simulink model "mcb_pmsm_foc_host_model_dyno_f28069m_Lab_2_GITHUB"  (R2023b)
settings: Solver=ode3  StartTime=0.0  StopTime=inf  RelTol=1e-3
undefined symbols (not defined in the file): PU_System_motor1, PU_System_motor2, Ts
libraries: instrumentseriallib x3, simulink x3, demo_controls x1
settings Model: Creator=The MathWorks, Inc.  LastModifiedBy=Jonathan
settings SolverCC: AlgebraicLoopSolver=TrustRegion  AutoInsertRateTranBlk=on  MaxZcPerStep=1
settings DataIOCC: LimitDataPoints=on  SaveFormat=Array  ReturnWorkspaceOutputs=off
settings OptimizationCC: LifeSpan=1  EfficientTunableParamExpr=on
settings DebuggingCC: UnderspecifiedInitializationDetection=Classic  MergeDetectMultiDrivingBlocksExec=none  SolverPrmCheckMsg=warning  ParameterPrecisionLossMsg=none  UnconnectedInputMsg=warning  UnconnectedOutputMsg=warning  UnconnectedLineMsg=warning  AllowSymbolicDim=off  PregeneratedLibrarySubsystemCodeDiagnostic=none  SFUnexpectedBacktrackingDiag=warning  SFNoUnconditionalDefaultTransitionDiag=warning  SFExecutionAtInitializationDiag=none  ArithmeticOperatorsInVariantConditions=warning
settings HardwareCC: ProdBitPerPointer=32  ProdLargestAtomicFloat=None  ProdIntDivRoundTo=Undefined  ProdEndianess=Unspecified  ProdWordSize=32  ProdHWDeviceType=32-bit Generic
settings ModelReferenceCC: EnableRefExpFcnMdlSchedulingChecks=on  PropagateSignalLabelsOutOfModel=off
settings SFSimCC: SimUseLocalCustomCode=off  MATLABDynamicMemAlloc=off
settings RTWCC: Description=Real-Time Workshop Embedded Coder  SystemTargetFile=ert.tlc  TemplateMakefile=ert_default_tmf  GenerateReport=on  RTWUseLocalCustomCode=off  IncludeHyperlinkInReport=on  LaunchReport=on  GenerateTraceInfo=on  GenerateTraceReport=on  GenerateTraceReportSl=on  GenerateTraceReportSf=on  GenerateTraceReportEml=on  DLArmComputeVersion=19.05
settings CodeAppCC: IgnoreCustomStorageClasses=off  StateflowObjectComments=on  InternalIdentifier=Classic
settings ERTTargetCC: MultiwordLength=2048  GenerateSampleERTMain=on  ERTCustomFileTemplate=example_file_process.tlc  ConvertIfToSwitch=off  SuppressUnreachableDefaultCases=off
settings ConfigComp: CovMetricSettings=dw  CovSaveCumulativeToWorkspaceVar=on  CovSaveSingleToWorkspaceVar=on  CovExternalEMLEnable=off  CovSFcnEnable=off

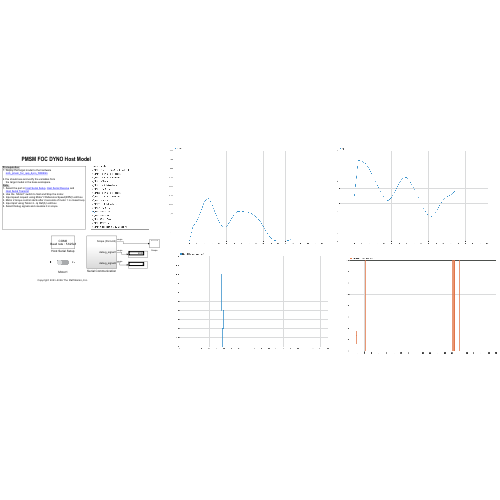
[thumbnail: Simulink's stored preview of the top-level diagram]
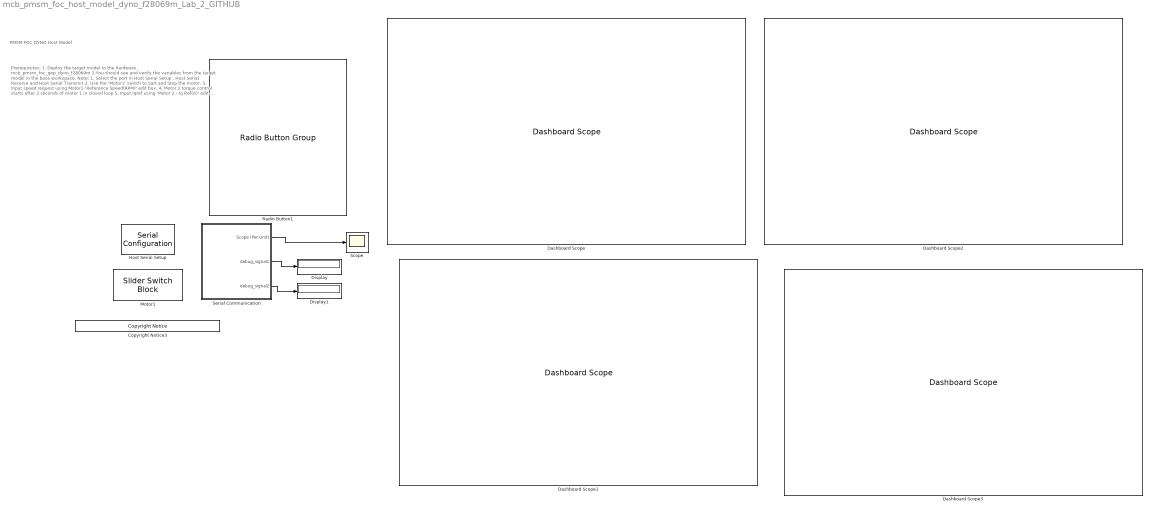
== system mcb_pmsm_foc_host_model_dyno_f28069m_Lab_2_GITHUB ==
  note: Prerequisites:
      | 1. Deploy the target model to the hardware
      | mcb_pmsm_foc_qep_dyno_f28069m
      |
      | 2.You should see and verify the variables from
      | the target model in the base workspace.
      | Note:
      | 1. Select the port in Host Serial Setup , Host Serial Receive and
      | Host Serial Transmit
      | 2. Use the 'Motor1' switch to Sart and Stop the motor.
      | 3. Input speed request using Motor1-'Reference Speed(RPM)' edit box.
      | 4. Motor 2 torque control starts after 2 seconds of motor 1 in closed loop
      | 5. Input Iqref using 'Motor 2 - Iq Ref(A)' edit box
      | 6. Select Debug signals and visualize it in scope.
  note: PMSM FOC DYNO Host Model
  Copyright Notice3 : demo_controls/Copyright Notice  year=2021  prod=tic2000
  Dashboard Scope : DashboardScope  TimeSpan=40  Ymin=-10  Ymax=5000  ScaleAtStop=off
  Dashboard Scope1 : DashboardScope  TimeSpan=100  Ymin=-0  Ymax=5  ScaleAtStop=off
  Dashboard Scope2 : DashboardScope  TimeSpan=40  Ymin=-6  Ymax=6  ScaleAtStop=off
  Dashboard Scope3 : DashboardScope  TimeSpan=40  Ymin=0  Ymax=4000  ScaleAtStop=off
  Display : Display
  Display1 : Display
  Host Serial Setup : instrumentseriallib/Serial Configuration  Priority=-99  PortSel=COM6  Port=COM6  ComPort=COM6  BaudRate=5.625e6  DataBits=8  Parity=none  StopBits=1  ByteOrder=little-endian  FlowControl=none  Timeout=2  SimulateUsing=Interpreted execution  BlockInModel=on  aMode=5
  Motor1 : SliderSwitchBlock  LabelPosition=Hide
      settings: Values={{'Stop', 'Start'}, [0 1]}
  Radio Button1 : RadioButtonGroup  LabelPosition=Hide  SelectedLabel=Mtr1&Mtr2: Pm  ButtonGroupName=Debug signals
      settings: Values={{'Mtr1: Speed ref & Speed feedback', 'Mtr1: Id ref & Id feedback', 'Mtr1: Iq ref & Iq feedback', 'Mtr1: Vd & Vq', 'Mtr1: Ia & Ib feedback', 'Mtr1: Pm & Te', 'Mtr2: Id ref & Id feedback', 'Mtr2: Iq ref & Iq feedback', 'Mtr2: Vd & Vq', 'Mtr2: Ia & Ib feedback', 'Mtr2: Pm & Te', 'Mtr1&Mtr2: Pm', 'Mtr1&Mtr2: Te', 'Mtr1&Mtr2: Pos', 'Mtr1&Mtr2: Ia', 'Mtr1 Speed ref & Mtr2 Speed fb'}, [1 2 3 4 5 6 7 8 9 10 11 12 13 14 15 0]}
  Scope : Scope
  Serial Communication : Subsystem
  wires:
  Serial Communication/1(Scope (Per-Unit)) -> Scope/1
  Serial Communication/2(debug_signal1) -> Display/1
  Serial Communication/3(debug_signal2) -> Display1/1

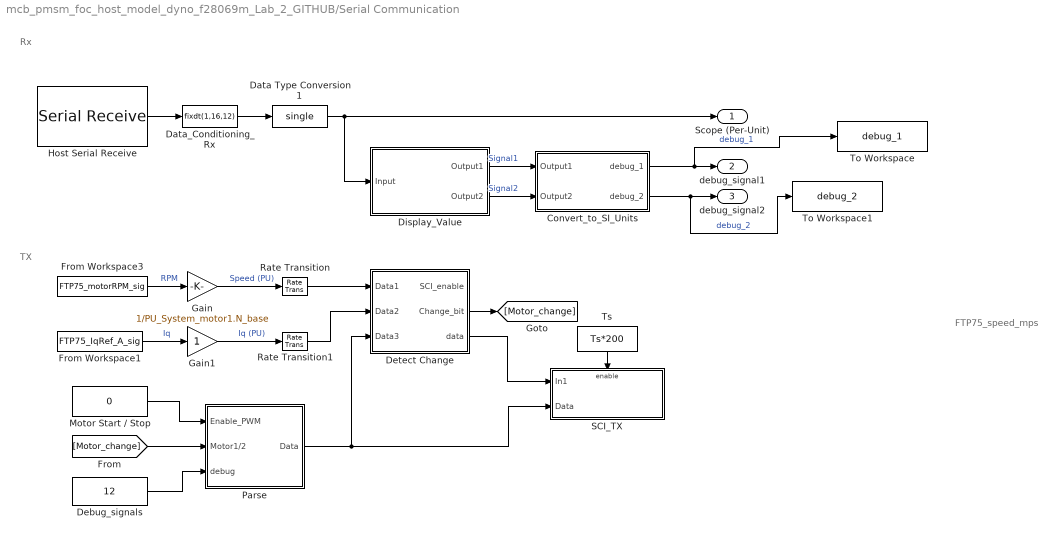
== system mcb_pmsm_foc_host_model_dyno_f28069m_Lab_2_GITHUB/Serial Communication ==
  note: FTP75_speed_mps
  note: TX
  note: Rx
  Convert_to_SI_Units : Subsystem
  Data Type Conversion1 : DataTypeConversion  OutDataTypeStr=single  RndMeth=Simplest  SaturateOnIntegerOverflow=off
  Data_Conditioning_Rx : DataTypeConversion  OutDataTypeStr=fixdt(1,16,12)  ConvertRealWorld=Stored Integer (SI)  RndMeth=Nearest
  Debug_signals : Constant  Value=12  OutDataTypeStr=uint16  SampleTime=0.03
  Detect Change : Subsystem
  Display_Value : MATLAB Function  TreatAsAtomicUnit=on
  From Workspace1 : FromWorkspace  VariableName=FTP75_IqRef_A_sig
  From Workspace3 : FromWorkspace  VariableName=FTP75_motorRPM_sig
  Gain : Gain  Gain=1/PU_System_motor1.N_base  OutDataTypeStr=single  RndMeth=Simplest
  Gain1 : Gain  RndMeth=Simplest  OutDataTypeStr=Inherit: Same as input
  Host Serial Receive : instrumentseriallib/Serial Receive  PortSel=COM6  Port=COM6  ComPort=COM6  DataType=uint16  SaveDataType=uint8  ToggleHeader=on  Header='SS'  DataSize=[600 2]  ToggleTerminator=on  Terminator=Custom terminator  CustomTerminator='EE'  InputFormat=Row major  ToggleDataSize=on  EnableBlockingMode=on  ActionDataUnavailable=Output last received value  ActionWhenDataUnavailable=Output last received value  CustomValue=0  SampleTime=Ts*200  SimulateUsing=Interpreted execution  BlockInModel=on  aMode=5
  Motor Start / Stop : Constant  Value=0  VectorParams1D=off  OutDataTypeStr=uint16  SampleTime=0.03
  Parse : Subsystem
  Rate Transition : RateTransition  OutPortSampleTime=0.03
  Rate Transition1 : RateTransition  OutPortSampleTime=0.03
  SCI_TX : Subsystem  TreatAsAtomicUnit=on
  To Workspace : ToWorkspace  VariableName=debug_1  SaveFormat=Timeseries  SampleTime=-1
  To Workspace1 : ToWorkspace  VariableName=debug_2  SaveFormat=Timeseries  SampleTime=-1
  Ts : Constant  Value=Ts*200  VectorParams1D=off  OutDataTypeStr=boolean  SampleTime=0.03
  Scope (Per-Unit) : Outport
  debug_signal1 : Outport  Port=2
  debug_signal2 : Outport  Port=3
  wires:
  Detect Change/2(Change_bit) -> [Motor_change]
  Gain/1 -> Rate Transition/1  "Speed (PU)"
  Motor Start / Stop/1 -> Parse/1(Enable_PWM)
  Parse/1(Data) -> SCI_TX/2(Data), Detect Change/3(Data3)
  Debug_signals/1 -> Parse/3(debug)
  Detect Change/3(data) -> SCI_TX/1(In1)
  Rate Transition1/1 -> Detect Change/2(Data2)
  Gain1/1 -> Rate Transition1/1  "Iq (PU)"
  Rate Transition/1 -> Detect Change/1(Data1)
  [Motor_change] -> Parse/2(Motor1/2)
  Host Serial Receive/1 -> Data_Conditioning_Rx/1
  Convert_to_SI_Units/2(debug_2) -> To Workspace1/1, debug_signal2/1  "debug_2"
  Convert_to_SI_Units/1(debug_1) -> To Workspace/1, debug_signal1/1  "debug_1"
  Data_Conditioning_Rx/1 -> Data Type Conversion1/1
  Display_Value/2(Output2) -> Convert_to_SI_Units/2(Output2)  "Signal2"
  Display_Value/1(Output1) -> Convert_to_SI_Units/1(Output1)  "Signal1"
  Data Type Conversion1/1 -> Scope (Per-Unit)/1, Display_Value/1(Input)
  Ts/1 -> SCI_TX/Enable
  From Workspace3/1 -> Gain/1  "RPM"
  From Workspace1/1 -> Gain1/1  "Iq"

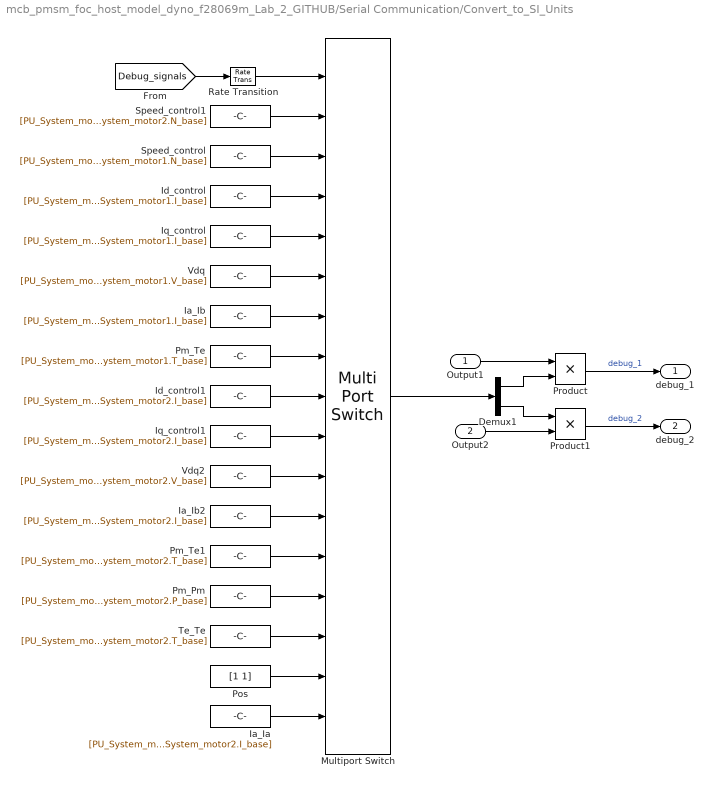
== system mcb_pmsm_foc_host_model_dyno_f28069m_Lab_2_GITHUB/Serial Communication/Convert_to_SI_Units ==
  Output1 : Inport
  Output2 : Inport  Port=2
  Demux1 : Demux  Outputs=2
  Ia_Ia : Constant  Value=[PU_System_motor1.I_base PU_System_motor2.I_base]  OutDataTypeStr=uint16  SampleTime=-1
  Ia_Ib : Constant  Value=[PU_System_motor1.I_base PU_System_motor1.I_base]  OutDataTypeStr=uint16  SampleTime=-1
  Ia_Ib2 : Constant  Value=[PU_System_motor2.I_base PU_System_motor2.I_base]  OutDataTypeStr=uint16  SampleTime=-1
  Id_control : Constant  Value=[PU_System_motor1.I_base PU_System_motor1.I_base]  OutDataTypeStr=uint16  SampleTime=-1
  Id_control1 : Constant  Value=[PU_System_motor2.I_base PU_System_motor2.I_base]  OutDataTypeStr=uint16  SampleTime=-1
  Iq_control : Constant  Value=[PU_System_motor1.I_base PU_System_motor1.I_base]  OutDataTypeStr=uint16  SampleTime=-1
  Iq_control1 : Constant  Value=[PU_System_motor2.I_base PU_System_motor2.I_base]  OutDataTypeStr=uint16  SampleTime=-1
  Multiport Switch : MultiPortSwitch  DataPortOrder=Zero-based contiguous  Inputs=16  DiagnosticForDefault=Warning  zeroidx=on  OutDataTypeStr=uint16  RndMeth=Simplest  SaturateOnIntegerOverflow=off  InputSameDT=off
  Pm_Pm : Constant  Value="[PU_System_motor1.P_base  PU_System_motor2.P_base]"  OutDataTypeStr=uint16  SampleTime=-1
  Pm_Te : Constant  Value="[PU_System_motor1.P_base  PU_System_motor1.T_base]"  OutDataTypeStr=uint16  SampleTime=-1
  Pm_Te1 : Constant  Value="[PU_System_motor2.P_base  PU_System_motor2.T_base]"  OutDataTypeStr=uint16  SampleTime=-1
  Pos : Constant  Value=[1 1]  OutDataTypeStr=uint16  SampleTime=-1
  Product : Product
  Product1 : Product
  Rate Transition : RateTransition  Deterministic=off
  Speed_control : Constant  Value=[PU_System_motor1.N_base PU_System_motor1.N_base]  OutDataTypeStr=uint16  SampleTime=-1
  Speed_control1 : Constant  Value=[PU_System_motor1.N_base PU_System_motor2.N_base]  OutDataTypeStr=uint16  SampleTime=-1
  Te_Te : Constant  Value="[PU_System_motor1.T_base  PU_System_motor2.T_base]"  OutDataTypeStr=uint16  SampleTime=-1
  Vdq : Constant  Value=[PU_System_motor1.V_base PU_System_motor1.V_base]  OutDataTypeStr=uint16  SampleTime=-1
  Vdq2 : Constant  Value=[PU_System_motor2.V_base PU_System_motor2.V_base]  OutDataTypeStr=uint16  SampleTime=-1
  debug_1 : Outport
  debug_2 : Outport  Port=2
  wires:
  Product/1 -> debug_1/1  "debug_1"
  Product1/1 -> debug_2/1  "debug_2"
  [Debug_signals] -> Rate Transition/1
  Multiport Switch/1 -> Demux1/1
  Demux1/1 -> Product/2
  Output1/1 -> Product/1
  Rate Transition/1 -> Multiport Switch/1
  Pos/1 -> Multiport Switch/16
  Ia_Ia/1 -> Multiport Switch/17
  Te_Te/1 -> Multiport Switch/15
  Pm_Pm/1 -> Multiport Switch/14
  Pm_Te1/1 -> Multiport Switch/13
  Ia_Ib2/1 -> Multiport Switch/12
  Vdq2/1 -> Multiport Switch/11
  Iq_control1/1 -> Multiport Switch/10
  Id_control1/1 -> Multiport Switch/9
  Pm_Te/1 -> Multiport Switch/8
  Ia_Ib/1 -> Multiport Switch/7
  Vdq/1 -> Multiport Switch/6
  Iq_control/1 -> Multiport Switch/5
  Id_control/1 -> Multiport Switch/4
  Speed_control/1 -> Multiport Switch/3
  Speed_control1/1 -> Multiport Switch/2
  Demux1/2 -> Product1/1
  Output2/1 -> Product1/2

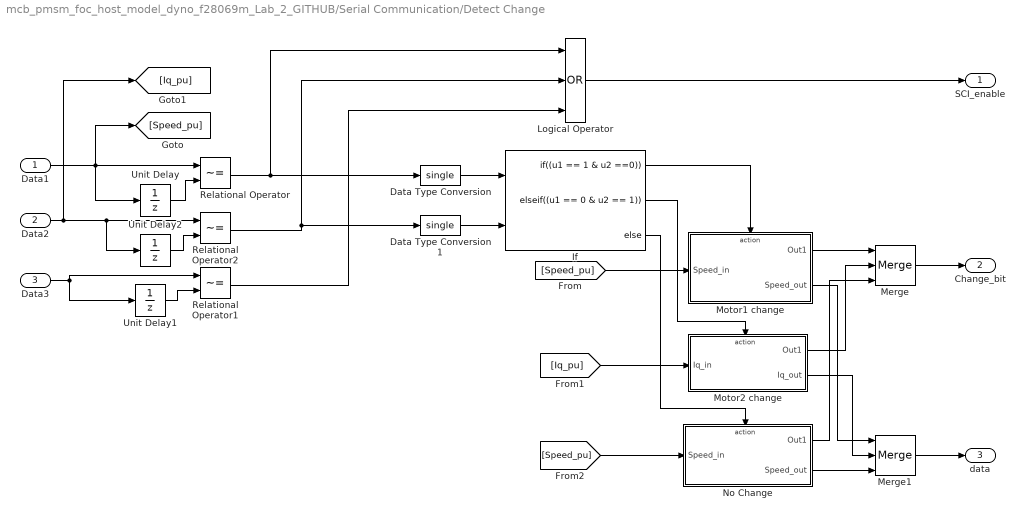
== system mcb_pmsm_foc_host_model_dyno_f28069m_Lab_2_GITHUB/Serial Communication/Detect Change ==
  Data1 : Inport
  Data2 : Inport  Port=2
  Data3 : Inport  Port=3
  Data Type Conversion : DataTypeConversion  OutDataTypeStr=single  SaturateOnIntegerOverflow=off  RndMeth=Floor
  Data Type Conversion1 : DataTypeConversion  OutDataTypeStr=single  SaturateOnIntegerOverflow=off  RndMeth=Floor
  If : If  NumInputs=2  IfExpression=(u1 == 1 & u2 ==0)  ElseIfExpressions=(u1 == 0 & u2 == 1)
  Logical Operator : Logic  Operator=OR  Inputs=3  AllPortsSameDT=off  OutDataTypeStr=boolean
  Merge : Merge  Inputs=3
  Merge1 : Merge  Inputs=3
  Motor1 change : Subsystem  TreatAsAtomicUnit=on
  Motor2 change : Subsystem  TreatAsAtomicUnit=on
  No Change : Subsystem  TreatAsAtomicUnit=on
  Relational Operator : RelationalOperator  Operator=~=  OutDataTypeStr=boolean  InputSameDT=off
  Relational Operator1 : RelationalOperator  Operator=~=  OutDataTypeStr=boolean  InputSameDT=off
  Relational Operator2 : RelationalOperator  Operator=~=  OutDataTypeStr=boolean  InputSameDT=off
  Unit Delay : UnitDelay  InitialCondition=0.5  SampleTime=-1  HasFrameUpgradeWarning=on
  Unit Delay1 : UnitDelay  SampleTime=-1  HasFrameUpgradeWarning=on
  Unit Delay2 : UnitDelay  InitialCondition=0.5  SampleTime=-1  HasFrameUpgradeWarning=on
  SCI_enable : Outport
  Change_bit : Outport  Port=2
  data : Outport  Port=3
  wires:
  Data1/1 -> [Speed_pu], Unit Delay/1, Relational Operator/1
  Unit Delay/1 -> Relational Operator/2
  Unit Delay2/1 -> Relational Operator2/2
  Data2/1 -> [Iq_pu], Unit Delay2/1, Relational Operator2/1
  Data3/1 -> Relational Operator1/1, Unit Delay1/1
  Logical Operator/1 -> SCI_enable/1
  Relational Operator2/1 -> Logical Operator/2, Data Type Conversion1/1
  Merge/1 -> Change_bit/1
  Relational Operator/1 -> Logical Operator/1, Data Type Conversion/1
  Motor2 change/1(Out1) -> Merge/2
  If/3 -> No Change/Action
  If/2 -> Motor2 change/Action
  No Change/1(Out1) -> Merge/3
  Merge1/1 -> data/1
  Motor2 change/2(Iq_out) -> Merge1/2
  No Change/2(Speed_out) -> Merge1/3
  Motor1 change/1(Out1) -> Merge/1
  Motor1 change/2(Speed_out) -> Merge1/1
  Data Type Conversion/1 -> If/1
  Data Type Conversion1/1 -> If/2
  If/1 -> Motor1 change/Action
  Unit Delay1/1 -> Relational Operator1/2
  Relational Operator1/1 -> Logical Operator/3
  [Speed_pu] -> Motor1 change/1(Speed_in)
  [Iq_pu] -> Motor2 change/1(Iq_in)
  [Speed_pu] -> No Change/1(Speed_in)

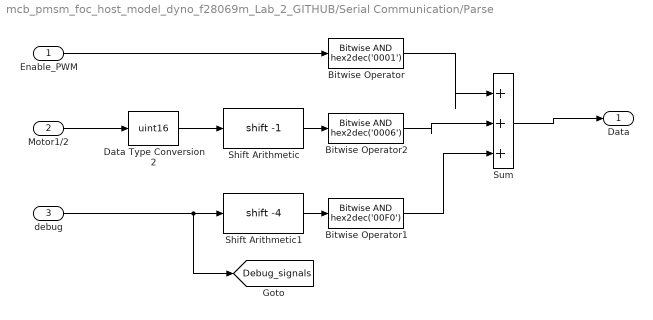
== system mcb_pmsm_foc_host_model_dyno_f28069m_Lab_2_GITHUB/Serial Communication/Parse ==
  Enable_PWM : Inport
  Motor1/2 : Inport  Port=2
  debug : Inport  Port=3
  Bitwise Operator : simulink/Logic and Bit Operations/Bitwise Operator  logicop=AND  UseBitMask=on  BitMask=hex2dec('0001')  BitMaskRealWorld=Stored Integer
  Bitwise Operator1 : simulink/Logic and Bit Operations/Bitwise Operator  logicop=AND  UseBitMask=on  BitMask=hex2dec('00F0')  BitMaskRealWorld=Stored Integer
  Bitwise Operator2 : simulink/Logic and Bit Operations/Bitwise Operator  logicop=AND  UseBitMask=on  BitMask=hex2dec('0006')  BitMaskRealWorld=Stored Integer
  Data Type Conversion2 : DataTypeConversion  OutDataTypeStr=uint16  SaturateOnIntegerOverflow=off  RndMeth=Floor
  Shift Arithmetic : ArithShift  BitShiftNumber=-1
  Shift Arithmetic1 : ArithShift  BitShiftNumber=-4
  Sum : Sum  Inputs=|+++
  Data : Outport
  tag scope: Debug_signals=global
  wires:
  Bitwise Operator/1 -> Sum/1
  Sum/1 -> Data/1
  Shift Arithmetic1/1 -> Bitwise Operator1/1
  Shift Arithmetic/1 -> Bitwise Operator2/1
  Bitwise Operator1/1 -> Sum/3
  Motor1/2/1 -> Data Type Conversion2/1
  Bitwise Operator2/1 -> Sum/2
  Enable_PWM/1 -> Bitwise Operator/1
  debug/1 -> [Debug_signals], Shift Arithmetic1/1
  Data Type Conversion2/1 -> Shift Arithmetic/1

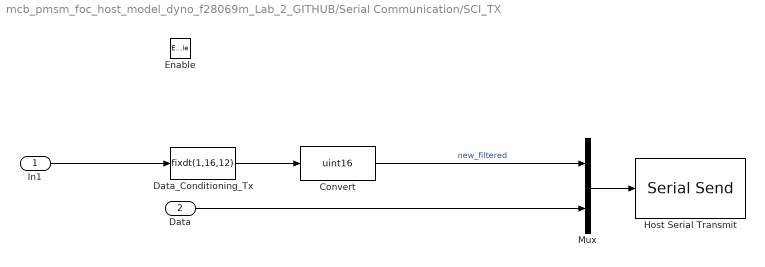
== system mcb_pmsm_foc_host_model_dyno_f28069m_Lab_2_GITHUB/Serial Communication/SCI_TX ==
  In1 : Inport
  Data : Inport  Port=2
  Enable : EnablePort
  Convert : DataTypeConversion  OutDataTypeStr=uint16  ConvertRealWorld=Stored Integer (SI)  RndMeth=Simplest  SaturateOnIntegerOverflow=off
  Data_Conditioning_Tx : DataTypeConversion  OutDataTypeStr=fixdt(1,16,12)  RndMeth=Simplest  SaturateOnIntegerOverflow=off
  Host Serial Transmit : instrumentseriallib/Serial Send  PortSel=COM6  Port=COM6  ComPort=COM6  Header=[]  Terminator=<none>  CustomTerminator=[]  EnableBlockingMode=off  SimulateUsing=Interpreted execution  BlockInModel=on  aMode=5
  Mux : Mux  Inputs=2
  wires:
  Data_Conditioning_Tx/1 -> Convert/1
  Mux/1 -> Host Serial Transmit/1
  Data/1 -> Mux/2
  In1/1 -> Data_Conditioning_Tx/1
  Convert/1 -> Mux/1  "new_filtered"

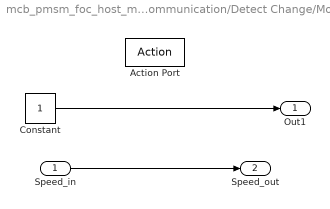
== system mcb_pmsm_foc_host_model_dyno_f28069m_Lab_2_GITHUB/Serial Communication/Detect Change/Motor1 change ==
  Speed_in : Inport
  Action Port : ActionPort  ActionPortLabel=if((u1 == 1 & u2 ==0))
  Constant : Constant  OutDataTypeStr=uint16
  Out1 : Outport  InitialOutput=1
  Speed_out : Outport  Port=2
  wires:
  Constant/1 -> Out1/1
  Speed_in/1 -> Speed_out/1

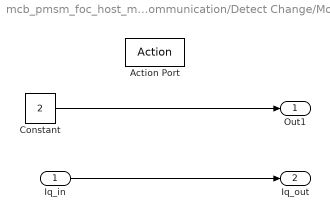
== system mcb_pmsm_foc_host_model_dyno_f28069m_Lab_2_GITHUB/Serial Communication/Detect Change/Motor2 change ==
  Iq_in : Inport
  Action Port : ActionPort  ActionPortLabel=elseif((u1 == 0 & u2 == 1))
  Constant : Constant  Value=2  OutDataTypeStr=uint16
  Out1 : Outport  InitialOutput=02
  Iq_out : Outport  Port=2
  wires:
  Constant/1 -> Out1/1
  Iq_in/1 -> Iq_out/1

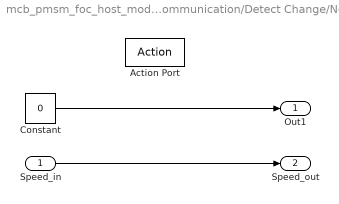
== system mcb_pmsm_foc_host_model_dyno_f28069m_Lab_2_GITHUB/Serial Communication/Detect Change/No Change ==
  Speed_in : Inport
  Action Port : ActionPort  ActionPortLabel=else
  Constant : Constant  Value=0  OutDataTypeStr=uint16
  Out1 : Outport  InitialOutput=0
  Speed_out : Outport  Port=2
  wires:
  Constant/1 -> Out1/1
  Speed_in/1 -> Speed_out/1

== matlab function mcb_pmsm_foc_host_model_dyno_f28069m_Lab_2_GITHUB/Serial Communication/Display_Value ==
  data: Output1 output; Input input; Output2 output
function [Output1, Output2] = unBuf (Input)
%% ************************************************************************
% Unbuffer function
% Outputs first received serial data from buffer for both signals

% Copyright 2020 The MathWorks, Inc.

selSignal= Input(:, 1);
Output1 = selSignal(1,1);
selSignal = Input(:, 2);
Output2 = selSignal(1,1);
end
